simulink model "model_GF"  (R2022b)
settings: Solver=VariableStepAuto  StartTime=0.0  StopTime=30  RelTol=1e-3
values from neighbouring files (symbols this model uses):
  C_f = (0.066*C_b)    (= 0.00220630670953)    [model_GF_code.m]
  f_b = 50    [model_GF_code.m]
  Kic = R_f/ti    (= 1.587)    [model_GF_code.m]
  Kpc = L_f/ti    [model_GF_code.m]
  L_f = V_dc/(24*f_sw*delta_IL_max)    [model_GF_code.m]
  L_g = 1*L_f    [model_GF_code.m]
  R_d = 0.2    [model_GF_code.m]
  R_f = 0.005*Z_b    (= 0.0004761)    [model_GF_code.m]
  R_g = 0.005*Z_b    (= 0.0004761)    [model_GF_code.m]
  S_b = 5e6    (= 5000000)    [model_GF_code.m]
  T_s = 100e-6    (= 0.0001)    [model_GF_code.m]
  V_dc = 3*V_m    [model_GF_code.m]
  w_c = 0.1*w_b    (= 31.4159265359)    [model_GF_code.m]
libraries: spsabctodq0Lib x6, spsThreePhaseSeriesRLCBranchLib x4, spsPowerdq0InstantaneousLib x3, spsThreePhaseVIMeasurementLib x3, slpidlib x2, spsGroundLib x2, spsPLL3phLib x2, spsdq0toabcLib x2, spsDCVoltageSourceLib x1, spsPWMGenerator2LevelLib x1, spsPower3phPhasorLib x1, simulink x1
settings Model: Creator=MSİ  LastModifiedBy=MSİ

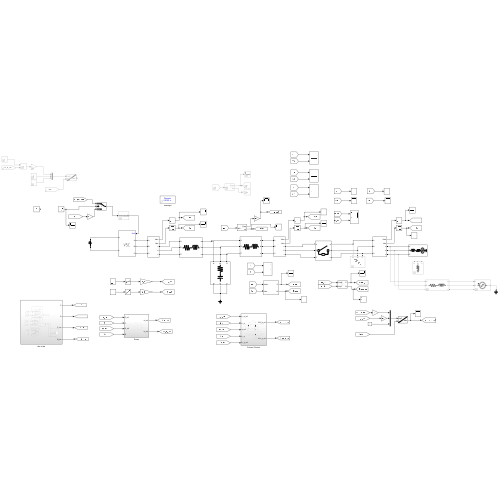
[thumbnail: Simulink's stored preview of the top-level diagram]
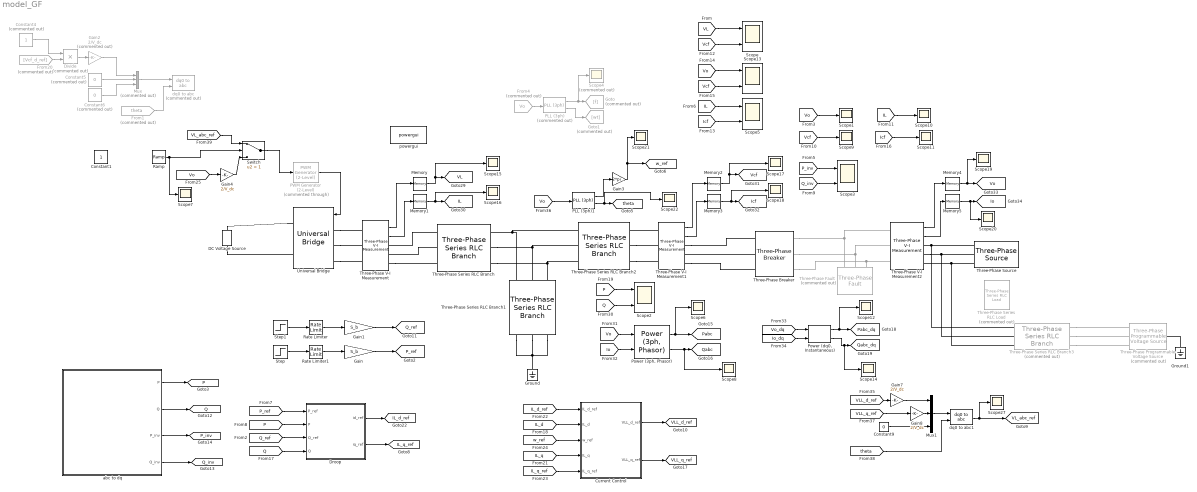
== system model_GF ==
  Constant1 : Constant
  Constant4 : Constant  Commented=on
  Constant5 : Constant  Commented=on  Value=0
  Constant6 : Constant  Commented=on  Value=0
  Constant9 : Constant  Value=0
  Current Control : Subsystem
  DC Voltage Source : spsDCVoltageSourceLib/DC Voltage Source  Amplitude=V_dc  Measurements=None
  Divide : Product  Commented=on  Inputs=**
  Droop : Subsystem
  From1 : From  Commented=on  GotoTag=theta  TagVisibility=global
  From20 : From  Commented=on  GotoTag=Vcf_d_ref  TagVisibility=global
  From4 : From  Commented=on  GotoTag=Vo  TagVisibility=global
  Gain : Gain  Gain=S_b
  Gain1 : Gain  Gain=S_b
  Gain2 : Gain  Commented=on  Gain=2/V_dc
  Gain3 : Gain  Gain=2*pi
  Gain4 : Gain  Gain=2/V_dc
  Gain7 : Gain  Gain=2/V_dc
  Gain8 : Gain  Gain=2/V_dc
  Goto : Goto  Commented=on  GotoTag=f
  Goto1 : Goto  Commented=on  GotoTag=wt
  Ground : spsGroundLib/Ground  LConnTagsString=a
  Ground1 : spsGroundLib/Ground  LConnTagsString=a
  Memory{,1..5} (6 alike) : Memory
  Mux : Mux  Commented=on  Inputs=3
  Mux1 : Mux  Inputs=3
  PLL (3ph) : spsPLL3phLib/PLL (3ph)  Commented=on  Fmin=45  Par_Init=[0, 50]  ParK=[180, 3200, 1]  TcD=1e-4  MaxRateChangeFreq=12  FilterCutOffFreq=25  Ts=0  AGC=on
  PLL (3ph)1 : spsPLL3phLib/PLL (3ph)  Fmin=45  Par_Init=[0, 50]  ParK=[180, 3200, 1]  TcD=1e-4  MaxRateChangeFreq=12  FilterCutOffFreq=25  Ts=0  AGC=on
  PWM Generator (2-Level) : spsPWMGenerator2LevelLib/PWM Generator (2-Level)  Commented=through  ModulatorType=Three-phase bridge (6 pulses)  ModulatorMode=Unsynchronized  Fc=5000  Pc=-90  nF=5000/50  MinMax="[ -1  1 ]"  SamplingTechnique=Natural  ModulatingSignals=off  m=2/V_dc  Freq=50  Phase=0  Ts=0  ShowCarrierOutport=off
  "Power (3ph, Phasor)" : spsPower3phPhasorLib/Power (3ph, Phasor)
      settings: LibrarySourceBlock=|
      | sps_lib/Sensors and Measurements/Power
      | (3ph, Phasor)
  "Power (dq0, Instantaneous)" : spsPowerdq0InstantaneousLib/Power (dq0, Instantaneous)
      settings: LibrarySourceBlock=|
      | sps_lib/Sensors and Measurements/Power
      | (dq0, Instantaneous)
  Ramp : simulink/Sources/Ramp  slope=1  start=0  InitialOutput=0
  Rate Limiter : RateLimiter  RisingSlewLimit=0.4  FallingSlewLimit=-0.2  SampleTimeMode=inherited
  Rate Limiter1 : RateLimiter  RisingSlewLimit=0.2  FallingSlewLimit=-0.1  SampleTimeMode=inherited
  Scope{,2..3,5,13} (5 alike) : Scope  NumInputPorts=2
  Scope{1,6..12,14..22,27} (18 alike) : Scope
  Scope4 : Scope  Commented=on
  Step : Step  Time=5  SampleTime=0
  Step1 : Step  Time=12  After=0.6  SampleTime=0
  Switch : Switch  Criteria=u2 > Threshold  Threshold=1  SaturateOnIntegerOverflow=off  InputSameDT=off
  Three-Phase Programmable Voltage Source : spsThreePhaseProgrammableVoltageSourceLib/Three-Phase Programmable Voltage Source  Commented=on  PositiveSequence="[690  0 50]"  VariationEntity=None  VariationType=Ramp  VariationTypeAlt=Ramp  VariationStep=0.5  VariationRate=0.05  VariationMagnitude=0.3  VariationFrequency=2  VariationTiming=[18 22]  VariationPhaseA=off  Amplitudes=[1 0.8 1.2 1.0]  TimeValues=[0 0.1 0.15 0.2]  HarmonicGeneration=off  HarmonicA=[3 0.2 -25 0]  HarmonicB=[2 0.15 35 2]  Timing="[0.05  3]"  BusType=swing  Pref=0  Qref=0  Qmin=-inf  Qmax=inf
  Three-Phase Series RLC Branch : spsThreePhaseSeriesRLCBranchLib/Three-Phase Series RLC Branch  LConnTagsString=A|B|C  RConnTagsString=A|B|C  BranchType=RL  Resistance=R_f  Inductance=L_f  Capacitance=1e-6  Measurements=None
  Three-Phase Series RLC Branch1 : spsThreePhaseSeriesRLCBranchLib/Three-Phase Series RLC Branch  LConnTagsString=A|B|C  RConnTagsString=A|B|C  BranchType=RC  Resistance=R_d  Inductance=1e-3  Capacitance=C_f  Measurements=None
  Three-Phase Series RLC Branch2 : spsThreePhaseSeriesRLCBranchLib/Three-Phase Series RLC Branch  LConnTagsString=A|B|C  RConnTagsString=A|B|C  BranchType=RL  Resistance=R_g  Inductance=L_g  Capacitance=1e-6  Measurements=None
  Three-Phase Series RLC Branch3 : spsThreePhaseSeriesRLCBranchLib/Three-Phase Series RLC Branch  Commented=on  LConnTagsString=A|B|C  RConnTagsString=A|B|C  BranchType=RL  Resistance=9.5e-4  Inductance=3e-5  Capacitance=1e-6  Measurements=None
  Three-Phase Series RLC Load : spsThreePhaseSeriesRLCLoadLib/Three-Phase Series RLC Load  Commented=on  LConnTagsString=A|B|C  Configuration=Y (grounded)  NominalVoltage=V_b  Vabc=[1e3 1e3 1e3]  Vabcp=[1e3 1e3 1e3]  NominalFrequency=50  UnbalancedPower=off  ActivePower=1e6  InductivePower=0  CapacitivePower=0  Pabc=[10e3 9e3 11e3]  QLabc=[100 90 110]  QCabc=[100 90 110]  Pabcp=[10e3 9e3 11e3]  QLabcp=[100 90 110]  QCabcp=[100 90 110]  Measurements=None  LoadType=constant Z
  Three-Phase V-I Measurement : spsThreePhaseVIMeasurementLib/Three-Phase V-I Measurement  VoltageMeasurement=phase-to-ground  SetLabelV=off  LabelV=VL  Vpu=off  VpuLL=off  CurrentMeasurement=yes  SetLabelI=off  LabelI=IL  Ipu=off  Pbase=100e6  Vbase=500e3  OutputType=Complex  PhasorSimulation=off  PSBequivalent=0
  Three-Phase V-I Measurement1 : spsThreePhaseVIMeasurementLib/Three-Phase V-I Measurement  VoltageMeasurement=phase-to-ground  SetLabelV=off  LabelV=Vcf  Vpu=off  VpuLL=off  CurrentMeasurement=yes  SetLabelI=off  LabelI=Icf  Ipu=off  Pbase=100e6  Vbase=500e3  OutputType=Complex  PhasorSimulation=off  PSBequivalent=0
  Three-Phase V-I Measurement2 : spsThreePhaseVIMeasurementLib/Three-Phase V-I Measurement  VoltageMeasurement=phase-to-ground  SetLabelV=off  LabelV=Vo  Vpu=off  VpuLL=off  CurrentMeasurement=yes  SetLabelI=off  LabelI=Io  Ipu=off  Pbase=100e6  Vbase=500e3  OutputType=Complex  PhasorSimulation=off  PSBequivalent=0
  Three-Phase Breaker : spsThreePhaseBreakerLib/Three-Phase Breaker  InitialState=open  SwitchA=on  SwitchB=on  SwitchC=on  SwitchTimes=[1]  External=off  BreakerResistance=0.01/5  SnubberResistance=1e6  SnubberCapacitance=inf  Measurements=None
  Three-Phase Fault : spsThreePhaseFaultLib/Three-Phase Fault  Commented=on  InitialStates=0  FaultA=on  FaultB=on  FaultC=on  GroundFault=on  SwitchTimes="[16  16.1]"  External=off  SwitchStatus=NaN  FaultResistance=0.001  GroundResistance=0.01  SnubberResistance=1e6  SnubberCapacitance=inf  Measurements=None
  Three-Phase Source : spsThreePhaseSourceLib/Three-Phase Source  InternalConnection=Yg  VoltagePhases=off  Voltage=(690)*1  PhaseAngle=0  Voltage_phases=[25e3 25e3 25e3]/sqrt(3)  PhaseAngles_phases=[0 -120 +120]  Frequency=f_b  NonIdealSource=on  SpecifyImpedance=on  Resistance=0.8929  Inductance=16.58e-3  ShortCircuitLevel=S_b*10  BaseVoltage=V_b  XRratio=10  BusType=swing  Pref=1000000  Qref=1000000  Prefabc=[10e3, 10e3, 10e3]  Qrefabc=[0, 0, 0]  Qmin=-Inf  Qmax=Inf
  Universal Bridge : spsUniversalBridgeLib/Universal Bridge  Arms=3  SnubberResistance=1e5  SnubberCapacitance=inf  Device=Average-model based VSC  Ron=1e-3  Lon=0  ForwardVoltages="[  0  0  ]"  ForwardVoltage=0  GTOparameters=[ 10e-6 , 20e-6 ]  IGBTparameters=[ 1e-6 , 2e-6 ]  Measurements=Device voltages  Measurements_2=None  converterType=Rectifier
  abc to dq : Subsystem
  dq0 to abc : spsdq0toabcLib/dq0 to abc  Commented=on  Alignment=90 degrees behind phase A axis
  dq0 to abc1 : spsdq0toabcLib/dq0 to abc  Alignment=90 degrees behind phase A axis
  powergui : spspowerguiLib/powergui  Priority=1  SimulationMode=Discrete  SampleTime=T_s  frequency=60  Iterations=50  frequencyindice=0  Pbase=100e6  ErrMax=1e-4  UnitsV=kV  UnitsW=MW  buscounter=0  FunctionMessages=off  echomessages=off  EnableUseOfTLC=off  CurrentSourceSwitches=off  DisableSnubberDevices=off  DisableRonSwitches=off  DisableVfSwitches=off  DisplayEquations=off  AutomaticDiscreteSolvers=off  SolverType=Tustin/Backward Euler (TBE)  Interpol=off  ExternalGateDelay=off  methode=off  Ts=100  x0status=blocks  SPID=on  SwTol=0  HookPort=off  NonlinearTolerance=1e-4  nMaxIteration=100  ContinueOnMaxIteration=off  RestoreLinks=warning  ResistiveCurrentMeasurement=off  Frange=[0:2:500]  Ylog=off  Xlog=on  ShowGrid=off  save=off  variable=ZData  structure=0  ZoomFFT=off  StartTime=0.0  cycles=1  DisplayStyle=1  fundamental=60  FreqAxis=off  MaxFrequency=1000  frequencyindicesteady=1  RmsSteady=1  display=off
  tag scope: IL=global, IL_d_ref=global, IL_q_ref=global, Icf=global, Io=global, P=global, P_inv=global, P_ref=global, Pabc=global, Pabc_dq=global, Q=global, Q_inv=global, Q_ref=global, Qabc=global, Qabc_dq=global, VL=global, VLL_d_ref=global, VLL_q_ref=global, VL_abc_ref=global, Vcf=global, Vo=global, theta=global, w_ref=global
  wires:
  [VL] -> Scope/1
  [Vo] -> Scope1/1
  From4/1 -> PLL (3ph)/1
  PLL (3ph)/1 -> Scope4/1, Goto/1
  PLL (3ph)/2 -> Goto1/1
  Constant5/1 -> Mux/2
  Constant6/1 -> Mux/3
  PWM Generator (2-Level)/1 -> Universal Bridge/1
  [IL] -> Scope5/1
  Step/1 -> Rate Limiter1/1
  Gain/1 -> [P_ref]
  [Vcf] -> Scope/2
  [Icf] -> Scope5/2
  [Vo] -> Scope13/1
  [Vcf] -> Scope13/2
  Gain1/1 -> [Q_ref]
  Step1/1 -> Rate Limiter/1
  Gain2/1 -> Mux/1
  From20/1 -> Divide/2
  Divide/1 -> Gain2/1
  Constant4/1 -> Divide/1
  [Vcf] -> Scope9/1
  [IL] -> Scope10/1
  [Icf] -> Scope11/1
  Constant9/1 -> Mux1/3
  Mux1/1 -> dq0 to abc1/1
  [theta] -> dq0 to abc1/2
  dq0 to abc1/1 -> Scope27/1, [VL_abc_ref]
  [VLL_d_ref] -> Gain7/1
  Gain7/1 -> Mux1/1
  Gain8/1 -> Mux1/2
  [VLL_q_ref] -> Gain8/1
  Mux/1 -> dq0 to abc/1
  From1/1 -> dq0 to abc/2
  [P_ref] -> Droop/1(P_ref)
  [P] -> Droop/2(P)
  [Q_ref] -> Droop/3(Q_ref)
  [Q] -> Droop/4(Q)
  Droop/2(iq_ref) -> [IL_q_ref]
  [IL_d_ref] -> Current Control/1(IL_d_ref)
  [IL_d] -> Current Control/2(IL_d)
  [w_ref] -> Current Control/3(w_ref)
  [IL_q] -> Current Control/4(IL_q)
  [IL_q_ref] -> Current Control/5(IL_q_ref)
  Current Control/1(VLL_d_ref) -> [VLL_d_ref]
  Current Control/2(VLL_q_ref) -> [VLL_q_ref]
  Memory/1 -> Scope15/1, [VL]
  Memory1/1 -> Scope16/1, [IL]
  Three-Phase V-I Measurement/1 -> Memory/1
  Three-Phase V-I Measurement/2 -> Memory1/1
  Memory3/1 -> Scope18/1, [Icf]
  Memory2/1 -> Scope17/1, [Vcf]
  Three-Phase V-I Measurement1/1 -> Memory2/1
  Three-Phase V-I Measurement1/2 -> Memory3/1
  Memory4/1 -> Scope19/1, [Vo]
  Memory5/1 -> Scope20/1, [Io]
  Three-Phase V-I Measurement2/1 -> Memory4/1
  Three-Phase V-I Measurement2/2 -> Memory5/1
  abc to dq/2(Q) -> [Q]
  abc to dq/1(P) -> [P]
  [P] -> Scope2/1
  [Q] -> Scope2/2
  abc to dq/3(P_inv) -> [P_inv]
  abc to dq/4(Q_inv) -> [Q_inv]
  [P_inv] -> Scope3/1
  [Q_inv] -> Scope3/2
  [Vo] -> "Power (3ph, Phasor)"/1
  [Io] -> "Power (3ph, Phasor)"/2
  "Power (3ph, Phasor)"/1 -> Scope6/1, [Pabc]
  "Power (3ph, Phasor)"/2 -> Scope8/1, [Qabc]
  [Vo_dq] -> "Power (dq0, Instantaneous)"/1
  [Io_dq] -> "Power (dq0, Instantaneous)"/2
  "Power (dq0, Instantaneous)"/1 -> Scope12/1, [Pabc_dq]
  "Power (dq0, Instantaneous)"/2 -> Scope14/1, [Qabc_dq]
  Rate Limiter/1 -> Gain1/1
  Rate Limiter1/1 -> Gain/1
  [Vo] -> PLL (3ph)1/1
  PLL (3ph)1/2 -> Scope22/1, [theta]
  Droop/1(id_ref) -> [IL_d_ref]
  PLL (3ph)1/1 -> Gain3/1
  Gain3/1 -> [w_ref], Scope21/1
  [Vo] -> Gain4/1
  Switch/1 -> PWM Generator (2-Level)/1
  Ramp/1 -> Scope7/1, Switch/2
  Gain4/1 -> Switch/3
  [VL_abc_ref] -> Switch/1
  connections:
  Universal Bridge/RConn1 -- DC Voltage Source/RConn1
  DC Voltage Source/LConn1 -- Universal Bridge/RConn2
  Three-Phase Series RLC Branch1/LConn1 -- Three-Phase Series RLC Branch2/LConn1 -- Three-Phase Series RLC Branch/RConn1
  Three-Phase Series RLC Branch/RConn2 -- Three-Phase Series RLC Branch2/LConn2 -- Three-Phase Series RLC Branch1/LConn2
  Three-Phase Series RLC Branch/RConn3 -- Three-Phase Series RLC Branch2/LConn3 -- Three-Phase Series RLC Branch1/LConn3
  Three-Phase Series RLC Branch1/RConn1 -- Three-Phase Series RLC Branch1/RConn3 -- Ground/LConn1 -- Three-Phase Series RLC Branch1/RConn2
  Three-Phase Series RLC Branch/LConn1 -- Three-Phase V-I Measurement/RConn1
  Three-Phase Series RLC Branch/LConn2 -- Three-Phase V-I Measurement/RConn2
  Universal Bridge/LConn1 -- Three-Phase V-I Measurement/LConn1
  Universal Bridge/LConn2 -- Three-Phase V-I Measurement/LConn2
  Universal Bridge/LConn3 -- Three-Phase V-I Measurement/LConn3
  Three-Phase V-I Measurement/RConn3 -- Three-Phase Series RLC Branch/LConn3
  Ground1/LConn1 -- Three-Phase Programmable Voltage Source/LConn1
  Three-Phase Fault/LConn1 -- Three-Phase V-I Measurement2/LConn1 -- Three-Phase Breaker/RConn1
  Three-Phase Fault/LConn2 -- Three-Phase V-I Measurement2/LConn2 -- Three-Phase Breaker/RConn2
  Three-Phase Fault/LConn3 -- Three-Phase V-I Measurement2/LConn3 -- Three-Phase Breaker/RConn3
  Three-Phase Series RLC Branch3/RConn1 -- Three-Phase Programmable Voltage Source/RConn1
  Three-Phase Series RLC Branch3/RConn2 -- Three-Phase Programmable Voltage Source/RConn2
  Three-Phase Series RLC Branch3/RConn3 -- Three-Phase Programmable Voltage Source/RConn3
  Three-Phase V-I Measurement2/RConn1 -- Three-Phase Series RLC Branch3/LConn1 -- Three-Phase Source/RConn1
  Three-Phase V-I Measurement2/RConn2 -- Three-Phase Series RLC Branch3/LConn2 -- Three-Phase Source/RConn2
  Three-Phase Source/RConn3 -- Three-Phase Series RLC Branch3/LConn3 -- Three-Phase V-I Measurement2/RConn3
  Three-Phase V-I Measurement1/LConn1 -- Three-Phase Series RLC Branch2/RConn1
  Three-Phase Series RLC Branch2/RConn2 -- Three-Phase V-I Measurement1/LConn2
  Three-Phase Series RLC Branch2/RConn3 -- Three-Phase V-I Measurement1/LConn3
  Three-Phase V-I Measurement1/RConn1 -- Three-Phase Breaker/LConn1
  Three-Phase Breaker/LConn2 -- Three-Phase V-I Measurement1/RConn2
  Three-Phase V-I Measurement1/RConn3 -- Three-Phase Breaker/LConn3

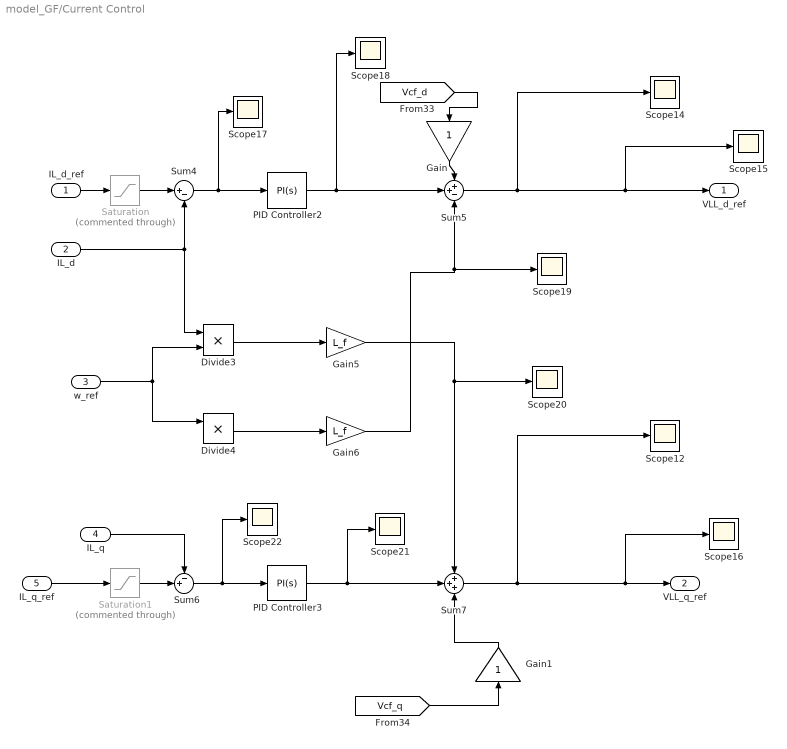
== system model_GF/Current Control ==
  IL_d_ref : Inport
  IL_d : Inport  Port=2
  w_ref : Inport  Port=3
  IL_q : Inport  Port=4
  IL_q_ref : Inport  Port=5
  Divide3 : Product  Inputs=**
  Divide4 : Product  Inputs=**
  Gain : Gain
  Gain1 : Gain
  Gain5 : Gain  Gain=L_f
  Gain6 : Gain  Gain=L_f
  PID Controller2 : slpidlib/PID Controller  Controller=PI  Form=Parallel  TimeDomain=Continuous-time  UseExternalTs=off  SampleTime=-1  IntegratorMethod=Forward Euler  FilterMethod=Forward Euler  ControllerParametersSource=internal  P=Kpc  I=Kic  UseKiTs=off  D=0  N=100  UseFilter=on  TunerSelectOption=Transfer Function Based (PID Tuner App)  InitialConditionSource=internal  InitialConditionForIntegrator=0  InitialConditionForFilter=0  DifferentiatorICPrevScaledInput=0  ExternalReset=none  TrackingMode=off  Kt=1  LimitOutput=off  SatLimitsSource=internal  UpperSaturationLimit=60  LowerSaturationLimit=-60  LinearizeAsGain=on  AntiWindupMode=none  Kb=1  LimitIntegrator=off  UpperIntegratorSaturationLimit=inf  LowerIntegratorSaturationLimit=-inf  POutMin=[]  POutMax=[]  IOutMin=[]  IOutMax=[]  DOutMin=[]  DOutMax=[]  NOutMin=[]  NOutMax=[]  SumOutMin=[]  SumOutMax=[]  SaturationOutMin=[]  SaturationOutMax=[]  PParamMin=[]  PParamMax=[]  IParamMin=[]  IParamMax=[]  DParamMin=[]  DParamMax=[]  NParamMin=[]  NParamMax=[]  KbParamMin=[]  KbParamMax=[]  KtParamMin=[]  KtParamMax=[]  KbOutMin=[]  KbOutMax=[]  KtOutMin=[]  KtOutMax=[]  IntegratorOutMin=[]  IntegratorOutMax=[]  FilterOutMin=[]  FilterOutMax=[]  SumI1OutMin=[]  SumI1OutMax=[]  SumI2OutMin=[]  SumI2OutMax=[]  SumI3OutMin=[]  SumI3OutMax=[]  SumI4OutMin=[]  SumI4OutMax=[]  SumDOutMin=[]  SumDOutMax=[]  DifferentiatorOutMin=[]  DifferentiatorOutMax=[]  FilterDiffOutCoefMin=[]  FilterDiffOutCoefMax=[]  ReciprocalOutMin=[]  ReciprocalOutMax=[]  SumDenOutMin=[]  SumDenOutMax=[]  SumNumOutMin=[]  SumNumOutMax=[]  DivideOutMin=[]  DivideOutMax=[]  UdiffTsProdOutMin=[]  UdiffTsProdOutMax=[]  NTsProdOutMin=[]  NTsProdOutMax=[]  UintegralTsProdOutMin=[]  UintegralTsProdOutMax=[]  UngainTsProdOutMin=[]  UngainTsProdOutMax=[]  ClampingZeroOutDataTypeStr=Inherit: Inherit via back propagation  ClampingZeroOutMin=[]  ClampingZeroOutMax=[]  FilterDenConstantOutDataTypeStr=Inherit: Inherit via back propagation  FilterDenConstantOutMin=[]  FilterDenConstantOutMax=[]  PCopyOutDataTypeStr=Inherit: Inherit via back propagation  PCopyOutMin=[]  PCopyOutMax=[]  NCopyOutDataTypeStr=Inherit: Inherit via back propagation  NCopyOutMin=[]  NCopyOutMax=[]  IntegratorContinuousStateAttributes=''  IntegratorStateMustResolveToSignalObject=off  IntegratorRTWStateStorageClass=Auto  FilterContinuousStateAttributes=''  FilterStateMustResolveToSignalObject=off  FilterRTWStateStorageClass=Auto  ParallelPVariant=InternalParameters  IdealPVariant=Disabled  IVariant=InternalParameters  DVariant=Disabled  IntegratorVariant=Continuous  SatVariant=Disabled  AWVariant=Passthrough  PCopyVariant=Disabled  TRVariant=Disabled  FdbkBlocksVariant=Forward  IdealPFdbkVariant=Disabled  SatFdbkVariant=Disabled  DerivativeFilterVariant=Disabled  NVariant=Disabled  NCopyVariant=Disabled_SignalSpec  FilterICVariant=Disabled  IntegratorICVariant=InternalICs  ExternalResetVariant=Disabled  TRSumVariant=Passthrough  SumFdbkVariant=Disabled  SumVariant=Sum_PI  TsampFilterVariant=InternalTs  TsampNgainVariant=Passthrough  TsampIntegralVariant=Passthrough  ExternalSaturationOutDataTypeStr=Inherit: Same as second input
  PID Controller3 : slpidlib/PID Controller  Controller=PI  Form=Parallel  TimeDomain=Continuous-time  UseExternalTs=off  SampleTime=-1  IntegratorMethod=Forward Euler  FilterMethod=Forward Euler  ControllerParametersSource=internal  P=Kpc  I=Kic  UseKiTs=off  D=0  N=100  UseFilter=on  TunerSelectOption=Transfer Function Based (PID Tuner App)  InitialConditionSource=internal  InitialConditionForIntegrator=0  InitialConditionForFilter=0  DifferentiatorICPrevScaledInput=0  ExternalReset=none  TrackingMode=off  Kt=1  LimitOutput=off  SatLimitsSource=internal  UpperSaturationLimit=26  LowerSaturationLimit=-20  LinearizeAsGain=on  AntiWindupMode=none  Kb=1  LimitIntegrator=off  UpperIntegratorSaturationLimit=inf  LowerIntegratorSaturationLimit=-inf  POutMin=[]  POutMax=[]  IOutMin=[]  IOutMax=[]  DOutMin=[]  DOutMax=[]  NOutMin=[]  NOutMax=[]  SumOutMin=[]  SumOutMax=[]  SaturationOutMin=[]  SaturationOutMax=[]  PParamMin=[]  PParamMax=[]  IParamMin=[]  IParamMax=[]  DParamMin=[]  DParamMax=[]  NParamMin=[]  NParamMax=[]  KbParamMin=[]  KbParamMax=[]  KtParamMin=[]  KtParamMax=[]  KbOutMin=[]  KbOutMax=[]  KtOutMin=[]  KtOutMax=[]  IntegratorOutMin=[]  IntegratorOutMax=[]  FilterOutMin=[]  FilterOutMax=[]  SumI1OutMin=[]  SumI1OutMax=[]  SumI2OutMin=[]  SumI2OutMax=[]  SumI3OutMin=[]  SumI3OutMax=[]  SumI4OutMin=[]  SumI4OutMax=[]  SumDOutMin=[]  SumDOutMax=[]  DifferentiatorOutMin=[]  DifferentiatorOutMax=[]  FilterDiffOutCoefMin=[]  FilterDiffOutCoefMax=[]  ReciprocalOutMin=[]  ReciprocalOutMax=[]  SumDenOutMin=[]  SumDenOutMax=[]  SumNumOutMin=[]  SumNumOutMax=[]  DivideOutMin=[]  DivideOutMax=[]  UdiffTsProdOutMin=[]  UdiffTsProdOutMax=[]  NTsProdOutMin=[]  NTsProdOutMax=[]  UintegralTsProdOutMin=[]  UintegralTsProdOutMax=[]  UngainTsProdOutMin=[]  UngainTsProdOutMax=[]  ClampingZeroOutDataTypeStr=Inherit: Inherit via back propagation  ClampingZeroOutMin=[]  ClampingZeroOutMax=[]  FilterDenConstantOutDataTypeStr=Inherit: Inherit via back propagation  FilterDenConstantOutMin=[]  FilterDenConstantOutMax=[]  PCopyOutDataTypeStr=Inherit: Inherit via back propagation  PCopyOutMin=[]  PCopyOutMax=[]  NCopyOutDataTypeStr=Inherit: Inherit via back propagation  NCopyOutMin=[]  NCopyOutMax=[]  IntegratorContinuousStateAttributes=''  IntegratorStateMustResolveToSignalObject=off  IntegratorRTWStateStorageClass=Auto  FilterContinuousStateAttributes=''  FilterStateMustResolveToSignalObject=off  FilterRTWStateStorageClass=Auto  ParallelPVariant=InternalParameters  IdealPVariant=Disabled  IVariant=InternalParameters  DVariant=Disabled  IntegratorVariant=Continuous  SatVariant=Disabled  AWVariant=Passthrough  PCopyVariant=Disabled  TRVariant=Disabled  FdbkBlocksVariant=Forward  IdealPFdbkVariant=Disabled  SatFdbkVariant=Disabled  DerivativeFilterVariant=Disabled  NVariant=Disabled  NCopyVariant=Disabled_SignalSpec  FilterICVariant=Disabled  IntegratorICVariant=InternalICs  ExternalResetVariant=Disabled  TRSumVariant=Passthrough  SumFdbkVariant=Disabled  SumVariant=Sum_PI  TsampFilterVariant=InternalTs  TsampNgainVariant=Passthrough  TsampIntegralVariant=Passthrough  ExternalSaturationOutDataTypeStr=Inherit: Same as second input
  Saturation : Saturate  Commented=through  UpperLimit=1.1*5500  LowerLimit=-1.1*5500
  Saturation1 : Saturate  Commented=through  UpperLimit=600  LowerLimit=-1.1*4500
  Scope{12,14..22} (10 alike) : Scope
  Sum4 : Sum  Inputs=|+-
  Sum5 : Sum  Inputs=++-
  Sum6 : Sum  Inputs=-+|
  Sum7 : Sum  Inputs=+++
  VLL_d_ref : Outport
  VLL_q_ref : Outport  Port=2
  wires:
  Sum5/1 -> VLL_d_ref/1, Scope15/1, Scope14/1
  Gain6/1 -> Scope19/1, Sum5/3
  Sum4/1 -> Scope17/1, PID Controller2/1
  PID Controller2/1 -> Scope18/1, Sum5/2
  PID Controller3/1 -> Scope21/1, Sum7/2
  Sum7/1 -> VLL_q_ref/1, Scope16/1, Scope12/1
  [Vcf_d] -> Gain/1
  Gain5/1 -> Scope20/1, Sum7/1
  Sum6/1 -> Scope22/1, PID Controller3/1
  Divide4/1 -> Gain6/1
  [Vcf_q] -> Gain1/1
  Divide3/1 -> Gain5/1
  IL_d_ref/1 -> Saturation/1
  IL_d/1 -> Sum4/2, Divide3/1
  w_ref/1 -> Divide4/1, Divide3/2
  IL_q/1 -> Sum6/1
  IL_q_ref/1 -> Saturation1/1
  Gain/1 -> Sum5/1
  Gain1/1 -> Sum7/3
  Saturation/1 -> Sum4/1
  Saturation1/1 -> Sum6/2

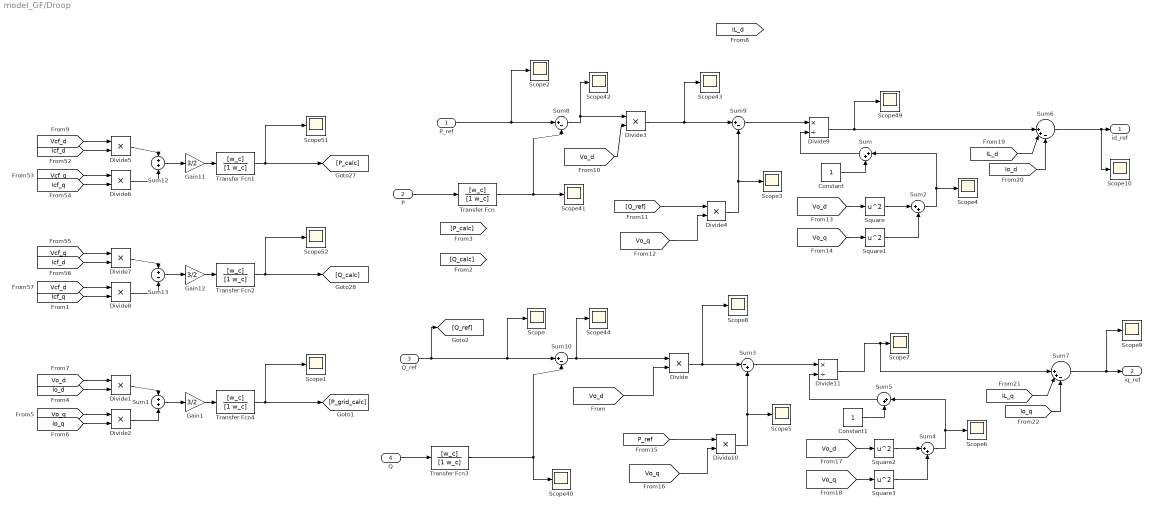
== system model_GF/Droop ==
  P_ref : Inport
  P : Inport  Port=2
  Q_ref : Inport  Port=3
  Q : Inport  Port=4
  Constant : Constant
  Constant1 : Constant
  Divide{,1..8,10} (10 alike) : Product  Inputs=**
  Divide11 : Product  Inputs=*/
  Divide9 : Product  Inputs=*/
  Gain1 : Gain  Gain=3/2
  Gain11 : Gain  Gain=3/2
  Gain12 : Gain  Gain=3/2
  Scope{,1..10,40..44,49,51..52} (19 alike) : Scope
  Square{,1..3} (4 alike) : Math  Operator=square
  Sum{,2,4..5} (4 alike) : Sum  Inputs=|++
  Sum1 : Sum  Inputs=+|+
  Sum10 : Sum  Inputs=|+-
  Sum12 : Sum  Inputs=+|+
  Sum13 : Sum  Inputs=+|-
  Sum3 : Sum  Inputs=|-+
  Sum6 : Sum  Inputs=||++-
  Sum7 : Sum  Inputs=||++-
  Sum8 : Sum  Inputs=|+-
  Sum9 : Sum  Inputs=|+-
  Transfer Fcn{,1..4} (5 alike) : TransferFcn  Numerator=[w_c]  Denominator=[1 w_c]
  id_ref : Outport
  iq_ref : Outport  Port=2
  wires:
  Sum8/1 -> Divide3/1, Scope42/1
  P_ref/1 -> Scope2/1, Sum8/1
  Q_ref/1 -> [Q_ref], Scope/1, Sum10/1
  Gain12/1 -> Transfer Fcn2/1
  Transfer Fcn1/1 -> Scope51/1, [P_calc]
  Transfer Fcn2/1 -> Scope52/1, [Q_calc]
  [Icf_d] -> Divide5/2
  Sum13/1 -> Gain12/1
  [Vcf_d] -> Divide8/1
  Divide5/1 -> Sum12/1
  [Vcf_q] -> Divide7/1
  [Icf_d] -> Divide7/2
  [Vcf_d] -> Divide5/1
  Divide8/1 -> Sum13/2
  [Vcf_q] -> Divide6/1
  [Icf_q] -> Divide6/2
  Gain11/1 -> Transfer Fcn1/1
  Sum12/1 -> Gain11/1
  Divide6/1 -> Sum12/2
  Divide7/1 -> Sum13/1
  [Icf_q] -> Divide8/2
  P/1 -> Transfer Fcn/1
  Q/1 -> Transfer Fcn3/1
  Transfer Fcn/1 -> Scope41/1, Sum8/2
  Transfer Fcn3/1 -> Sum10/2, Scope40/1
  Divide2/1 -> Sum1/2
  [Vo_q] -> Divide2/1
  Divide1/1 -> Sum1/1
  [Vo_d] -> Divide1/1
  Sum1/1 -> Gain1/1
  Transfer Fcn4/1 -> Scope1/1, [P_grid_calc]
  Gain1/1 -> Transfer Fcn4/1
  [Io_q] -> Divide2/2
  [Io_d] -> Divide1/2
  Divide3/1 -> Sum9/1, Scope43/1
  Divide/1 -> Scope8/1, Sum3/1
  Sum10/1 -> Divide/1, Scope44/1
  [Vo_d] -> Divide3/2
  [Vo_d] -> Divide/2
  Divide4/1 -> Scope3/1, Sum9/2
  [Q_ref] -> Divide4/1
  [Vo_q] -> Divide4/2
  Sum9/1 -> Divide9/1
  Divide9/1 -> Sum6/1, Scope49/1
  [Vo_d] -> Square/1
  [Vo_q] -> Square1/1
  Square/1 -> Sum2/1
  Square1/1 -> Sum2/2
  Sum2/1 -> Sum/1, Scope4/1
  Divide10/1 -> Sum3/2, Scope5/1
  [Vo_q] -> Divide10/2
  [P_ref] -> Divide10/1
  Square3/1 -> Sum4/2
  Sum3/1 -> Divide11/1
  Square2/1 -> Sum4/1
  Divide11/1 -> Sum7/1, Scope7/1
  Sum4/1 -> Sum5/1, Scope6/1
  [Vo_q] -> Square3/1
  [Vo_d] -> Square2/1
  Sum/1 -> Divide9/2
  Constant/1 -> Sum/2
  Constant1/1 -> Sum5/2
  Sum5/1 -> Divide11/2
  Sum6/1 -> Scope10/1, id_ref/1
  [IL_d] -> Sum6/2
  [Io_d] -> Sum6/3
  [IL_q] -> Sum7/2
  [Io_q] -> Sum7/3
  Sum7/1 -> Scope9/1, iq_ref/1

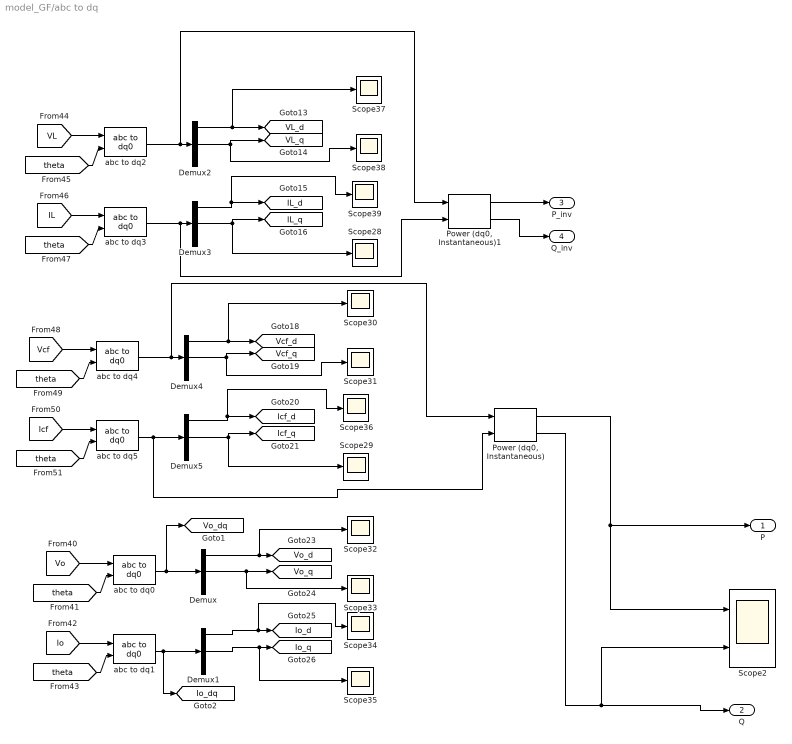
== system model_GF/abc to dq ==
  Demux{,1..5} (6 alike) : Demux  Outputs=3
  "Power (dq0, Instantaneous)" : spsPowerdq0InstantaneousLib/Power (dq0, Instantaneous)
      settings: LibrarySourceBlock=|
      | sps_lib/Sensors and Measurements/Power
      | (dq0, Instantaneous)
  "Power (dq0, Instantaneous)1" : spsPowerdq0InstantaneousLib/Power (dq0, Instantaneous)
      settings: LibrarySourceBlock=|
      | sps_lib/Sensors and Measurements/Power
      | (dq0, Instantaneous)
  Scope2 : Scope  NumInputPorts=2
  Scope{28..39} (12 alike) : Scope
  abc to dq{0..5} (6 alike) : spsabctodq0Lib/abc to dq0  Alignment=90 degrees behind phase A axis
  P : Outport
  Q : Outport  Port=2
  P_inv : Outport  Port=3
  Q_inv : Outport  Port=4
  tag scope: IL_d=global, IL_q=global, Icf_d=global, Icf_q=global, Io_d=global, Io_dq=global, Io_q=global, VL_d=global, VL_q=global, Vcf_d=global, Vcf_q=global, Vo_d=global, Vo_dq=global, Vo_q=global
  wires:
  [IL] -> abc to dq3/1
  Demux2/1 -> Scope37/1, [VL_d]
  abc to dq4/1 -> "Power (dq0, Instantaneous)"/1, Demux4/1
  Demux1/1 -> Scope34/1, [Io_d]
  abc to dq1/1 -> [Io_dq], Demux1/1
  Demux5/1 -> Scope36/1, [Icf_d]
  Demux2/2 -> Scope38/1, [VL_q]
  abc to dq0/1 -> [Vo_dq], Demux/1
  Demux/2 -> Scope33/1, [Vo_q]
  "Power (dq0, Instantaneous)"/1 -> Scope2/1, P/1
  Demux4/1 -> Scope30/1, [Vcf_d]
  Demux/1 -> Scope32/1, [Vo_d]
  "Power (dq0, Instantaneous)"/2 -> Scope2/2, Q/1
  [theta] -> abc to dq2/2
  [theta] -> abc to dq3/2
  [VL] -> abc to dq2/1
  [Vcf] -> abc to dq4/1
  abc to dq5/1 -> "Power (dq0, Instantaneous)"/2, Demux5/1
  [theta] -> abc to dq4/2
  Demux4/2 -> Scope31/1, [Vcf_q]
  [theta] -> abc to dq0/2
  Demux3/2 -> Scope28/1, [IL_q]
  Demux3/1 -> Scope39/1, [IL_d]
  abc to dq3/1 -> "Power (dq0, Instantaneous)1"/2, Demux3/1
  Demux1/2 -> Scope35/1, [Io_q]
  [theta] -> abc to dq1/2
  abc to dq2/1 -> "Power (dq0, Instantaneous)1"/1, Demux2/1
  Demux5/2 -> Scope29/1, [Icf_q]
  [theta] -> abc to dq5/2
  [Icf] -> abc to dq5/1
  [Io] -> abc to dq1/1
  [Vo] -> abc to dq0/1
  "Power (dq0, Instantaneous)1"/1 -> P_inv/1
  "Power (dq0, Instantaneous)1"/2 -> Q_inv/1
